simulink model "PPS_Scenario_003_cs"  (Simulink 7.6)
settings: Solver=ode5  SolverMode=SingleTasking  StartTime=0.0  StopTime=inf  FixedStep=1/100  RelTol=1e-3
model workspace (MAT data in the model file):
  mbox_table : struct (value not decoded)
  model_closed = 0
  sim_status = 0
PreLoadFcn:
  | check_NUTS_defined;
  | 
  | assignin('base',['model_closed_' bdroot],false);
  | 
  | addpath('../includes_PPS');
  | 
  | if exist('PPS_Model_sfun.mexw64')==3
  | delete PPS_Model_sfun.mexw64;
  | end
  | 
  | if exist('PPS_Model_sfun.mexw32') ==3
  | delete PPS_Model_sfun.mexw32;
  | end
  | 
  | switch version('-release')
  | case {'2010a', '2010b', '2011a'}
  | addpath('../includes_PPS/ML2010a');
  | case {'2011b', '2012a', '2012b'}
  | addpath('../includes_PPS/ML2011b');
  | otherwise
  | addpath('../includes_PPS/ML2011b');
  | end
InitFcn:
  | PreScanExperimentInitFcn(bdroot)
StopFcn:
  | PreScanExperimentStopFcn(bdroot)
undefined symbols (not defined in the file): DiscIntNeverNeededParam, InitImageOutputDir, x_ini_VRML, y_ini_VRML, z_ini_VRML
libraries: PreScanSimulinkLibrary x48, simulink x27, PreScanUsefulBlocks x20, simulink_extras x9, simulink_need_slupdate x1
(part 1 of 14)
CloseFcn:
  | evalin('base',['clear model_closed_' bdroot]);
settings Model: Creator=PRESCAN  LastModifiedBy=buildbot
settings DataIOCC: LimitDataPoints=off  MaxDataPoints=1  SaveOutput=off  SignalLogging=off  DSMLogging=off
settings OptimizationCC: InitFltsAndDblsToZero=on
settings DebuggingCC: SaveWithParameterizedLinksMsg=none  SignalResolutionControl=TryResolveAllWithWarning  SolverPrmCheckMsg=none  MultiTaskDSMMsg=warning  MultiTaskCondExecSysMsg=none  MultiTaskRateTransMsg=warning  UnknownTsInhSupMsg=none
settings SFSimCC: SimParseCustomCode=off
settings RTWCC: IncludeERTFirstTime=on
settings GRTTargetCC: TargetFcnLib=ansi_tfl_tmw.mat

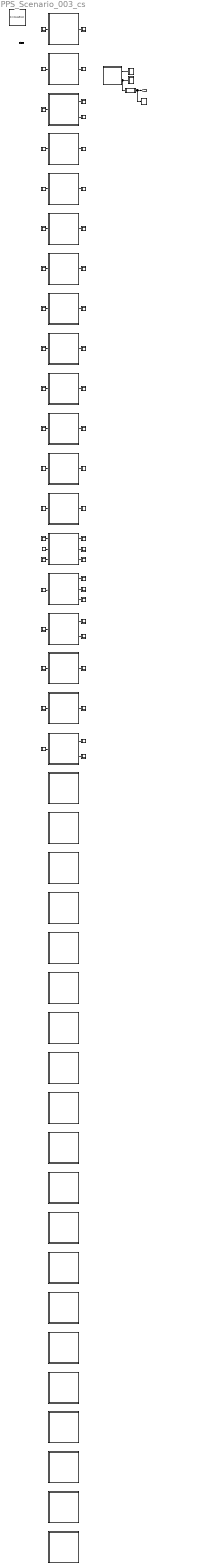
== system PPS_Scenario_003_cs ==
  note: OBU-Beacon ID
  note: Demo Help
  note: Regenerate
  note: Record for Replay
  note: Open Useful Blocks
  note: PreScan Options
  note: Version:
  note: 7.4.0
  note: Author(s):
  note: N.A.
  note: Descriptive text:
  note: ID
      |
      | 1
      | 8
      | 11
      | 16
      | 12
      | 19
      | 31
      | 47
      | 48
      | 49
      | 73
      | 93
      | 4
      | 7
      | 32
      | 66
      | 67
      | 68
      | 65
      | 15
      | 76
      | 10
      | 3
      | 78
      | 77
      | 79
      | 80
      | 81
      | 82
      | 83
      | 84
      | 85
      | 86
      | 89
      | 90
      | 92
      | 94
      | 95
      | 96
      | 103
      | 104
      | 105
      | 106
      | 114
      | 115
      | 57
      | 53
      | 58
      | 70
      | 97
      | 99
      | 100
      | 110
      | 108
      | 109
      | 112
  note: OBU-Beacon ID
  note: TypeID
      |
      | 1
      | 1
      | 1
      | 3
      | 4
      | 1
      | 1
      | 1
      | 1
      | 1
      | 3
      | 1
      | 1
      | 1
      | 1
      | 1
      | 7
      | 5
      | 1
      | 14
      | 14
      | 12
      | 12
      | 15
      | 15
      | 15
      | 15
      | 15
      | 15
      | 15
      | 15
      | 15
      | 15
      | 15
      | 15
      | 15
      | 15
      | 15
      | 15
      | 15
      | 15
      | 15
      | 15
      | 15
      | 15
      | 13
      | 13
      | 13
      | 13
      | 13
      | 13
      | 13
      | 13
      | 13
      | 13
      | 13
  note: TypeTag
      |
      | Car
      | Car
      | Car
      | Truck\Bus
      | Human
      | Car
      | Car
      | Car
      | Car
      | Car
      | Truck\Bus
      | Car
      | Car
      | Car
      | Car
      | Car
      | Unknown
      | Cal element
      | Car
      | Traffic sign
      | Traffic sign
      | Building
      | Building
      | Anim traffic sign
      | Anim traffic sign
      | Anim traffic sign
      | Anim traffic sign
      | Anim traffic sign
      | Anim traffic sign
      | Anim traffic sign
      | Anim traffic sign
      | Anim traffic sign
      | Anim traffic sign
      | Anim traffic sign
      | Anim traffic sign
      | Anim traffic sign
      | Anim traffic sign
      | Anim traffic sign
      | Anim traffic sign
      | Anim traffic sign
      | Anim traffic sign
      | Anim traffic sign
      | Anim traffic sign
      | Anim traffic sign
      | Anim traffic sign
      | Natural element
      | Natural element
      | Natural element
      | Natural element
      | Natural element
      | Natural element
      | Natural element
      | Natural element
      | Natural element
      | Natural element
      | Natural element
  note: SD
      |
      | Y
      | Y
      | Y
      | Y
      | Y
      | Y
      | Y
      | Y
      | Y
      | Y
      | Y
      | N
      | N
      | N
      | Y
      | Y
      | Y
      | Y
      | Y
      | Y
      | Y
      | Y
      | Y
      | Y
      | N
      | Y
      | Y
      | Y
      | Y
      | Y
      | Y
      | N
      | N
      | Y
      | Y
      | Y
      | Y
      | Y
      | Y
      | N
      | N
      | N
      | N
      | Y
      | Y
      | Y
      | Y
      | Y
      | Y
      | Y
      | Y
      | Y
      | Y
      | Y
      | Y
      | Y
  note: CD
      |
      | N
      | N
      | N
      | N
      | Y
      | N
      | N
      | N
      | N
      | N
      | N
      | N
      | N
      | Y
      | N
      | N
      | N
      | N
      | N
      | N
      | N
      | N
      | N
      | N
      | N
      | N
      | N
      | N
      | N
      | N
      | N
      | N
      | N
      | N
      | N
      | N
      | N
      | N
      | N
      | N
      | N
      | N
      | N
      | N
      | N
      | N
      | N
      | N
      | N
      | N
      | N
      | N
      | N
      | N
      | N
      | N
  note: Name
      |
      | BMW_X5_1
      | BMW_Z3_1
      | Toyota_Previa_1
      | Nissan_Cabstar_1
      | HumanAnimated_1
      | Mazda_RX8_2
      | Fiat_Bravo_2
      | Toyota_Previa_2
      | Toyota_Previa_3
      | Mazda_RX8_3
      | Nissan_Cabstar_2
      | Toyota_Previa_4
      | BMW_X5_2
      | Audi_A8_1
      | Toyota_Yaris_1
      | Ford_Fiesta_1
      | CarTrailer_SingleAxle_1
      | Sphere_1
      | Fiat_Bravo_1
      | TrafficSignPoleD_1
      | TrafficSignPoleD_2
      | OfficeBrownFlat_1
      | Busstop_1
      | Lightpost_2
      | Lightpost_1
      | Lightpost_3
      | Lightpost_4
      | Lightpost_5
      | Lightpost_6
      | Lightpost_7
      | Lightpost_8
      | Lightpost_9
      | Lightpost_10
      | InformationBoard_1
      | InformationBoard_2
      | Lightpost_11
      | Lightpost_12
      | Lightpost_13
      | Lightpost_14
      | Lightpost_15
      | Lightpost_16
      | Lightpost_17
      | Lightpost_18
      | Lightpost_19
      | Lightpost_20
      | TurkishHazel_Age20_5
      | TurkishHazel_Age10_1
      | TurkishHazel_Age10_2
      | TurkishHazel_Age20_1
      | TurkishHazel_Age20_6
      | TurkishHazel_Age20_8
      | TurkishHazel_Age20_9
      | TurkishHazel_Age20_13
      | TurkishHazel_Age20_10
      | TurkishHazel_Age20_11
      | TurkishHazel_Age20_12
  note: Num ID OBU-Beacon ID Type ID Type Tag SD CD Name
  Actuators : DataStoreMemory  Tag=Actuators  DataStoreName=SimCoreActuators  InitialValue=zeros(572,1)
      settings: DeleteFcn=PreScanBlockDeleteFcn;
  Audi_A8_1 : Subsystem  Tag=WorldObjectSubSystem  InitFcn=UniqueId = '210';
      mask Display: image(imread('Audi_A8.jpg'));color('white');text(0,0,' ID=7\n')
  BMW_X5_1 : Subsystem  Tag=WorldObjectSubSystem  InitFcn=UniqueId = '19';
      mask Display: image(imread('BMW_X5.jpg'));color('white');text(0,0,' ID=1\n')
  BMW_X5_2 : Subsystem  Tag=WorldObjectSubSystem  InitFcn=UniqueId = '173';
      mask Display: image(imread('BMW_X5.jpg'));color('white');text(0,0,' ID=4\n')
  BMW_Z3_1 : Subsystem  Tag=WorldObjectSubSystem  InitFcn=UniqueId = '21';
      mask Display: image(imread('BMW_Z3.jpg'));color('white');text(0,0,' ID=8\n')
  CameraSensor_1 : Subsystem  Tag=CameraSensor  Priority=3
      settings: DeleteFcn=PreScanBlockDeleteFcn;
      mask Type: PreScan Source Block: Camera Sensor
      mask Description: The Camera Sensor provides a color or monochrome image.
      mask Help: eval('openHelp(457)')
      mask Display: image(imread('CameraSensor.png'))
  CarTrailer_SingleAxle_1 : Subsystem  Tag=WorldObjectSubSystem  InitFcn=UniqueId = '232';
      mask Display: image(imread('CarTrailer_SingleAxle.jpg'));color('white');text(0,0,' ID=67\n')
  CollisionDetection : Subsystem  Tag=CollisionDetection  Priority=3  mask(PreScan Source Block: CollisionDetection){PortName=CollisionDetection, PortIndex=0, PortWidth=10, TimeStep=1/100}
      mask prompts: PortName "Auto-Assigned: Port Name [-]"; PortIndex "Auto-Assigned: Port Index [-]"; PortWidth "Auto-Assigned: Port Dimensions"; TimeStep "Auto-Assigned: Upload Period [s]"
      mask help:
      | The SELF port shows (state) information of the actor itself. The outputs are position in the experiment's axis system and the GPS coordinates, and the object's absolute velocity and compass heading.
      |
      | For more information, please click Help.
      settings: DeleteFcn=PreScanBlockDeleteFcn;
      mask Help: eval('openHelp(811)')
      mask Display: image(imread('crash.jpg'))
  Fiat_Bravo_1 : Subsystem  Tag=WorldObjectSubSystem  InitFcn=UniqueId = '271';
      mask Display: image(imread('Fiat_Bravo.jpg'));color('white');text(0,0,' ID=65\n')
  Fiat_Bravo_2 : Subsystem  Tag=WorldObjectSubSystem  InitFcn=UniqueId = '139';
      mask Display: image(imread('Fiat_Bravo.jpg'));color('white');text(0,0,' ID=31\n')
  Ford_Fiesta_1 : Subsystem  Tag=WorldObjectSubSystem  InitFcn=UniqueId = '231';
      mask Display: image(imread('Ford_Fiesta.jpg'));color('white');text(0,0,' ID=66\n')
  GetSensors : Subsystem  Tag=GetSensors  Priority=2  mask(PreScan Simulation Core Block){NrOfSensors=162, TimeStep=1/100}
      mask prompts: NrOfSensors "Number of sensor values"; TimeStep "Timestep [s]"
      mask help:
      | Please do not remove this block from the PreScan compilation sheet,
      | as it contains essential configuration parameters for a PreScan simulation.
      settings: DeleteFcn=PreScanBlockDeleteFcn;
  HumanAnimated_1 : Subsystem  Tag=WorldObjectSubSystem  InitFcn=UniqueId = '71';
      mask Display: image(imread('HumanTextured.jpg'));color('white');text(0,0,' ID=12\n')
  Lightpost_1 : Subsystem  Tag=WorldObjectSubSystem  InitFcn=UniqueId = '149';
      mask Display: image(imread('Lightpost.jpg'));color('white');text(0,0,' ID=77\n')
  Lightpost_10 : Subsystem  Tag=WorldObjectSubSystem  InitFcn=UniqueId = '157';
      mask Display: image(imread('Lightpost.jpg'));color('white');text(0,0,' ID=86\n')
  Lightpost_11 : Subsystem  Tag=WorldObjectSubSystem  InitFcn=UniqueId = '254';
      mask Display: image(imread('Lightpost.jpg'));color('white');text(0,0,' ID=92\n')
  Lightpost_12 : Subsystem  Tag=WorldObjectSubSystem  InitFcn=UniqueId = '256';
      mask Display: image(imread('Lightpost.jpg'));color('white');text(0,0,' ID=94\n')
  Lightpost_13 : Subsystem  Tag=WorldObjectSubSystem  InitFcn=UniqueId = '257';
      mask Display: image(imread('Lightpost.jpg'));color('white');text(0,0,' ID=95\n')
  Lightpost_14 : Subsystem  Tag=WorldObjectSubSystem  InitFcn=UniqueId = '258';
      mask Display: image(imread('Lightpost.jpg'));color('white');text(0,0,' ID=96\n')
  Lightpost_15 : Subsystem  Tag=WorldObjectSubSystem  InitFcn=UniqueId = '274';
      mask Display: image(imread('Lightpost.jpg'));color('white');text(0,0,' ID=103\n')
  Lightpost_16 : Subsystem  Tag=WorldObjectSubSystem  InitFcn=UniqueId = '275';
      mask Display: image(imread('Lightpost.jpg'));color('white');text(0,0,' ID=104\n')
  Lightpost_17 : Subsystem  Tag=WorldObjectSubSystem  InitFcn=UniqueId = '276';
      mask Display: image(imread('Lightpost.jpg'));color('white');text(0,0,' ID=105\n')
  Lightpost_18 : Subsystem  Tag=WorldObjectSubSystem  InitFcn=UniqueId = '277';
      mask Display: image(imread('Lightpost.jpg'));color('white');text(0,0,' ID=106\n')
  Lightpost_19 : Subsystem  Tag=WorldObjectSubSystem  InitFcn=UniqueId = '290';
      mask Display: image(imread('Lightpost.jpg'));color('white');text(0,0,' ID=114\n')
  Lightpost_2 : Subsystem  Tag=WorldObjectSubSystem  InitFcn=UniqueId = '148';
      mask Display: image(imread('Lightpost.jpg'));color('white');text(0,0,' ID=78\n')
  Lightpost_20 : Subsystem  Tag=WorldObjectSubSystem  InitFcn=UniqueId = '291';
      mask Display: image(imread('Lightpost.jpg'));color('white');text(0,0,' ID=115\n')
  Lightpost_3 : Subsystem  Tag=WorldObjectSubSystem  InitFcn=UniqueId = '150';
      mask Display: image(imread('Lightpost.jpg'));color('white');text(0,0,' ID=79\n')
  Lightpost_4 : Subsystem  Tag=WorldObjectSubSystem  InitFcn=UniqueId = '151';
      mask Display: image(imread('Lightpost.jpg'));color('white');text(0,0,' ID=80\n')
  Lightpost_5 : Subsystem  Tag=WorldObjectSubSystem  InitFcn=UniqueId = '152';
      mask Display: image(imread('Lightpost.jpg'));color('white');text(0,0,' ID=81\n')
  Lightpost_6 : Subsystem  Tag=WorldObjectSubSystem  InitFcn=UniqueId = '153';
      mask Display: image(imread('Lightpost.jpg'));color('white');text(0,0,' ID=82\n')
  Lightpost_7 : Subsystem  Tag=WorldObjectSubSystem  InitFcn=UniqueId = '154';
      mask Display: image(imread('Lightpost.jpg'));color('white');text(0,0,' ID=83\n')
  Lightpost_8 : Subsystem  Tag=WorldObjectSubSystem  InitFcn=UniqueId = '155';
      mask Display: image(imread('Lightpost.jpg'));color('white');text(0,0,' ID=84\n')
  Lightpost_9 : Subsystem  Tag=WorldObjectSubSystem  InitFcn=UniqueId = '156';
      mask Display: image(imread('Lightpost.jpg'));color('white');text(0,0,' ID=85\n')
  Mazda_RX8_2 : Subsystem  Tag=WorldObjectSubSystem  InitFcn=UniqueId = '114';
      mask Display: image(imread('Mazda_RX8.jpg'));color('white');text(0,0,' ID=19\n')
  Mazda_RX8_3 : Subsystem  Tag=WorldObjectSubSystem  InitFcn=UniqueId = '143';
      mask Display: image(imread('Mazda_RX8.jpg'));color('white');text(0,0,' ID=49\n')
  Nissan_Cabstar_1 : Subsystem  Tag=WorldObjectSubSystem  InitFcn=UniqueId = '45';
      mask Display: image(imread('Nissan_Cabstar.jpg'));color('white');text(0,0,' ID=16\n')
  Nissan_Cabstar_2 : Subsystem  Tag=WorldObjectSubSystem  InitFcn=UniqueId = '144';
      mask Display: image(imread('Nissan_Cabstar.jpg'));color('white');text(0,0,' ID=73\n')
  SELF_Audi_A8_1 : Subsystem  Tag=SELF  Priority=3  mask(PreScan Source Block: SELF){PortName=SELF_Audi_A8_1, PortIndex=114, PortWidth=8, TimeStep=1/100}
      mask prompts: PortName "Auto-Assigned: Port Name [-]"; PortIndex "Auto-Assigned: Port Index [-]"; PortWidth "Auto-Assigned: Port Dimensions"; TimeStep "Auto-Assigned: Upload Period [s]"
      mask help:
      | The SELF port shows (state) information of the actor itself. The outputs are position in the experiment's axis system and the GPS coordinates, and the object's absolute velocity and compass heading.
      |
      | For more information, please click Help.
      settings: DeleteFcn=PreScanBlockDeleteFcn;
      mask Help: eval('openHelp(462)')
      mask Display: image(imread('GPS.png'))
  SELF_BMW_X5_1 : Subsystem  Tag=SELF  Priority=3  mask(PreScan Source Block: SELF){PortName=SELF_BMW_X5_1, PortIndex=10, PortWidth=8, TimeStep=1/100}
      mask prompts: PortName "Auto-Assigned: Port Name [-]"; PortIndex "Auto-Assigned: Port Index [-]"; PortWidth "Auto-Assigned: Port Dimensions"; TimeStep "Auto-Assigned: Upload Period [s]"
      mask help:
      | The SELF port shows (state) information of the actor itself. The outputs are position in the experiment's axis system and the GPS coordinates, and the object's absolute velocity and compass heading.
      |
      | For more information, please click Help.
      settings: DeleteFcn=PreScanBlockDeleteFcn;
      mask Help: eval('openHelp(462)')
      mask Display: image(imread('GPS.png'))
  SELF_BMW_X5_2 : Subsystem  Tag=SELF  Priority=3  mask(PreScan Source Block: SELF){PortName=SELF_BMW_X5_2, PortIndex=106, PortWidth=8, TimeStep=1/100}
      mask prompts: PortName "Auto-Assigned: Port Name [-]"; PortIndex "Auto-Assigned: Port Index [-]"; PortWidth "Auto-Assigned: Port Dimensions"; TimeStep "Auto-Assigned: Upload Period [s]"
      mask help:
      | The SELF port shows (state) information of the actor itself. The outputs are position in the experiment's axis system and the GPS coordinates, and the object's absolute velocity and compass heading.
      |
      | For more information, please click Help.
      settings: DeleteFcn=PreScanBlockDeleteFcn;
      mask Help: eval('openHelp(462)')
      mask Display: image(imread('GPS.png'))
  SELF_BMW_Z3_1 : Subsystem  Tag=SELF  Priority=3  mask(PreScan Source Block: SELF){PortName=SELF_BMW_Z3_1, PortIndex=18, PortWidth=8, TimeStep=1/100}
      mask prompts: PortName "Auto-Assigned: Port Name [-]"; PortIndex "Auto-Assigned: Port Index [-]"; PortWidth "Auto-Assigned: Port Dimensions"; TimeStep "Auto-Assigned: Upload Period [s]"
      mask help:
      | The SELF port shows (state) information of the actor itself. The outputs are position in the experiment's axis system and the GPS coordinates, and the object's absolute velocity and compass heading.
      |
      | For more information, please click Help.
      settings: DeleteFcn=PreScanBlockDeleteFcn;
      mask Help: eval('openHelp(462)')
      mask Display: image(imread('GPS.png'))
  SELF_CarTrailer_SingleAxle_1 : Subsystem  Tag=SELF  Priority=3  mask(PreScan Source Block: SELF){PortName=SELF_CarTrailer_SingleAxle_1, PortIndex=138, PortWidth=8, TimeStep=1/100}
      mask prompts: PortName "Auto-Assigned: Port Name [-]"; PortIndex "Auto-Assigned: Port Index [-]"; PortWidth "Auto-Assigned: Port Dimensions"; TimeStep "Auto-Assigned: Upload Period [s]"
      mask help:
      | The SELF port shows (state) information of the actor itself. The outputs are position in the experiment's axis system and the GPS coordinates, and the object's absolute velocity and compass heading.
      |
      | For more information, please click Help.
      settings: DeleteFcn=PreScanBlockDeleteFcn;
      mask Help: eval('openHelp(462)')
      mask Display: image(imread('GPS.png'))
  SELF_Fiat_Bravo_1 : Subsystem  Tag=SELF  Priority=3  mask(PreScan Source Block: SELF){PortName=SELF_Fiat_Bravo_1, PortIndex=154, PortWidth=8, TimeStep=1/100}
      mask prompts: PortName "Auto-Assigned: Port Name [-]"; PortIndex "Auto-Assigned: Port Index [-]"; PortWidth "Auto-Assigned: Port Dimensions"; TimeStep "Auto-Assigned: Upload Period [s]"
      mask help:
      | The SELF port shows (state) information of the actor itself. The outputs are position in the experiment's axis system and the GPS coordinates, and the object's absolute velocity and compass heading.
      |
      | For more information, please click Help.
      settings: DeleteFcn=PreScanBlockDeleteFcn;
      mask Help: eval('openHelp(462)')
      mask Display: image(imread('GPS.png'))
  SELF_Fiat_Bravo_2 : Subsystem  Tag=SELF  Priority=3  mask(PreScan Source Block: SELF){PortName=SELF_Fiat_Bravo_2, PortIndex=58, PortWidth=8, TimeStep=1/100}
      mask prompts: PortName "Auto-Assigned: Port Name [-]"; PortIndex "Auto-Assigned: Port Index [-]"; PortWidth "Auto-Assigned: Port Dimensions"; TimeStep "Auto-Assigned: Upload Period [s]"
      mask help:
      | The SELF port shows (state) information of the actor itself. The outputs are position in the experiment's axis system and the GPS coordinates, and the object's absolute velocity and compass heading.
      |
      | For more information, please click Help.
      settings: DeleteFcn=PreScanBlockDeleteFcn;
      mask Help: eval('openHelp(462)')
      mask Display: image(imread('GPS.png'))
  SELF_Ford_Fiesta_1 : Subsystem  Tag=SELF  Priority=3  mask(PreScan Source Block: SELF){PortName=SELF_Ford_Fiesta_1, PortIndex=130, PortWidth=8, TimeStep=1/100}
      mask prompts: PortName "Auto-Assigned: Port Name [-]"; PortIndex "Auto-Assigned: Port Index [-]"; PortWidth "Auto-Assigned: Port Dimensions"; TimeStep "Auto-Assigned: Upload Period [s]"
      mask help:
      | The SELF port shows (state) information of the actor itself. The outputs are position in the experiment's axis system and the GPS coordinates, and the object's absolute velocity and compass heading.
      |
      | For more information, please click Help.
      settings: DeleteFcn=PreScanBlockDeleteFcn;
      mask Help: eval('openHelp(462)')
      mask Display: image(imread('GPS.png'))
  SELF_HumanAnimated_1 : Subsystem  Tag=SELF  Priority=3  mask(PreScan Source Block: SELF){PortName=SELF_HumanAnimated_1, PortIndex=42, PortWidth=8, TimeStep=1/100}
      mask prompts: PortName "Auto-Assigned: Port Name [-]"; PortIndex "Auto-Assigned: Port Index [-]"; PortWidth "Auto-Assigned: Port Dimensions"; TimeStep "Auto-Assigned: Upload Period [s]"
      mask help:
      | The SELF port shows (state) information of the actor itself. The outputs are position in the experiment's axis system and the GPS coordinates, and the object's absolute velocity and compass heading.
      |
      | For more information, please click Help.
      settings: DeleteFcn=PreScanBlockDeleteFcn;
      mask Help: eval('openHelp(462)')
      mask Display: image(imread('GPS.png'))
  SELF_Mazda_RX8_2 : Subsystem  Tag=SELF  Priority=3  mask(PreScan Source Block: SELF){PortName=SELF_Mazda_RX8_2, PortIndex=50, PortWidth=8, TimeStep=1/100}
      mask prompts: PortName "Auto-Assigned: Port Name [-]"; PortIndex "Auto-Assigned: Port Index [-]"; PortWidth "Auto-Assigned: Port Dimensions"; TimeStep "Auto-Assigned: Upload Period [s]"
      mask help:
      | The SELF port shows (state) information of the actor itself. The outputs are position in the experiment's axis system and the GPS coordinates, and the object's absolute velocity and compass heading.
      |
      | For more information, please click Help.
      settings: DeleteFcn=PreScanBlockDeleteFcn;
      mask Help: eval('openHelp(462)')
      mask Display: image(imread('GPS.png'))
  SELF_Mazda_RX8_3 : Subsystem  Tag=SELF  Priority=3  mask(PreScan Source Block: SELF){PortName=SELF_Mazda_RX8_3, PortIndex=82, PortWidth=8, TimeStep=1/100}
      mask prompts: PortName "Auto-Assigned: Port Name [-]"; PortIndex "Auto-Assigned: Port Index [-]"; PortWidth "Auto-Assigned: Port Dimensions"; TimeStep "Auto-Assigned: Upload Period [s]"
      mask help:
      | The SELF port shows (state) information of the actor itself. The outputs are position in the experiment's axis system and the GPS coordinates, and the object's absolute velocity and compass heading.
      |
      | For more information, please click Help.
      settings: DeleteFcn=PreScanBlockDeleteFcn;
      mask Help: eval('openHelp(462)')
      mask Display: image(imread('GPS.png'))
  SELF_Nissan_Cabstar_1 : Subsystem  Tag=SELF  Priority=3  mask(PreScan Source Block: SELF){PortName=SELF_Nissan_Cabstar_1, PortIndex=34, PortWidth=8, TimeStep=1/100}
      mask prompts: PortName "Auto-Assigned: Port Name [-]"; PortIndex "Auto-Assigned: Port Index [-]"; PortWidth "Auto-Assigned: Port Dimensions"; TimeStep "Auto-Assigned: Upload Period [s]"
      mask help:
      | The SELF port shows (state) information of the actor itself. The outputs are position in the experiment's axis system and the GPS coordinates, and the object's absolute velocity and compass heading.
      |
      | For more information, please click Help.
      settings: DeleteFcn=PreScanBlockDeleteFcn;
      mask Help: eval('openHelp(462)')
      mask Display: image(imread('GPS.png'))
  SELF_Nissan_Cabstar_2 : Subsystem  Tag=SELF  Priority=3  mask(PreScan Source Block: SELF){PortName=SELF_Nissan_Cabstar_2, PortIndex=90, PortWidth=8, TimeStep=1/100}
      mask prompts: PortName "Auto-Assigned: Port Name [-]"; PortIndex "Auto-Assigned: Port Index [-]"; PortWidth "Auto-Assigned: Port Dimensions"; TimeStep "Auto-Assigned: Upload Period [s]"
      mask help:
      | The SELF port shows (state) information of the actor itself. The outputs are position in the experiment's axis system and the GPS coordinates, and the object's absolute velocity and compass heading.
      |
      | For more information, please click Help.
      settings: DeleteFcn=PreScanBlockDeleteFcn;
      mask Help: eval('openHelp(462)')
      mask Display: image(imread('GPS.png'))
  SELF_Sphere_1 : Subsystem  Tag=SELF  Priority=3  mask(PreScan Source Block: SELF){PortName=SELF_Sphere_1, PortIndex=146, PortWidth=8, TimeStep=1/100}
      mask prompts: PortName "Auto-Assigned: Port Name [-]"; PortIndex "Auto-Assigned: Port Index [-]"; PortWidth "Auto-Assigned: Port Dimensions"; TimeStep "Auto-Assigned: Upload Period [s]"
      mask help:
      | The SELF port shows (state) information of the actor itself. The outputs are position in the experiment's axis system and the GPS coordinates, and the object's absolute velocity and compass heading.
      |
      | For more information, please click Help.
      settings: DeleteFcn=PreScanBlockDeleteFcn;
      mask Help: eval('openHelp(462)')
      mask Display: image(imread('GPS.png'))
  SELF_Toyota_Previa_1 : Subsystem  Tag=SELF  Priority=3  mask(PreScan Source Block: SELF){PortName=SELF_Toyota_Previa_1, PortIndex=26, PortWidth=8, TimeStep=1/100}
      mask prompts: PortName "Auto-Assigned: Port Name [-]"; PortIndex "Auto-Assigned: Port Index [-]"; PortWidth "Auto-Assigned: Port Dimensions"; TimeStep "Auto-Assigned: Upload Period [s]"
      mask help:
      | The SELF port shows (state) information of the actor itself. The outputs are position in the experiment's axis system and the GPS coordinates, and the object's absolute velocity and compass heading.
      |
      | For more information, please click Help.
      settings: DeleteFcn=PreScanBlockDeleteFcn;
      mask Help: eval('openHelp(462)')
      mask Display: image(imread('GPS.png'))
  SELF_Toyota_Previa_2 : Subsystem  Tag=SELF  Priority=3  mask(PreScan Source Block: SELF){PortName=SELF_Toyota_Previa_2, PortIndex=66, PortWidth=8, TimeStep=1/100}
      mask prompts: PortName "Auto-Assigned: Port Name [-]"; PortIndex "Auto-Assigned: Port Index [-]"; PortWidth "Auto-Assigned: Port Dimensions"; TimeStep "Auto-Assigned: Upload Period [s]"
      mask help:
      | The SELF port shows (state) information of the actor itself. The outputs are position in the experiment's axis system and the GPS coordinates, and the object's absolute velocity and compass heading.
      |
      | For more information, please click Help.
      settings: DeleteFcn=PreScanBlockDeleteFcn;
      mask Help: eval('openHelp(462)')
      mask Display: image(imread('GPS.png'))
  SELF_Toyota_Previa_3 : Subsystem  Tag=SELF  Priority=3  mask(PreScan Source Block: SELF){PortName=SELF_Toyota_Previa_3, PortIndex=74, PortWidth=8, TimeStep=1/100}
      mask prompts: PortName "Auto-Assigned: Port Name [-]"; PortIndex "Auto-Assigned: Port Index [-]"; PortWidth "Auto-Assigned: Port Dimensions"; TimeStep "Auto-Assigned: Upload Period [s]"
      mask help:
      | The SELF port shows (state) information of the actor itself. The outputs are position in the experiment's axis system and the GPS coordinates, and the object's absolute velocity and compass heading.
      |
      | For more information, please click Help.
      settings: DeleteFcn=PreScanBlockDeleteFcn;
      mask Help: eval('openHelp(462)')
      mask Display: image(imread('GPS.png'))
  SELF_Toyota_Previa_4 : Subsystem  Tag=SELF  Priority=3  mask(PreScan Source Block: SELF){PortName=SELF_Toyota_Previa_4, PortIndex=98, PortWidth=8, TimeStep=1/100}
      mask prompts: PortName "Auto-Assigned: Port Name [-]"; PortIndex "Auto-Assigned: Port Index [-]"; PortWidth "Auto-Assigned: Port Dimensions"; TimeStep "Auto-Assigned: Upload Period [s]"
      mask help:
      | The SELF port shows (state) information of the actor itself. The outputs are position in the experiment's axis system and the GPS coordinates, and the object's absolute velocity and compass heading.
      |
      | For more information, please click Help.
      settings: DeleteFcn=PreScanBlockDeleteFcn;
      mask Help: eval('openHelp(462)')
      mask Display: image(imread('GPS.png'))
  SELF_Toyota_Yaris_1 : Subsystem  Tag=SELF  Priority=3  mask(PreScan Source Block: SELF){PortName=SELF_Toyota_Yaris_1, PortIndex=122, PortWidth=8, TimeStep=1/100}
      mask prompts: PortName "Auto-Assigned: Port Name [-]"; PortIndex "Auto-Assigned: Port Index [-]"; PortWidth "Auto-Assigned: Port Dimensions"; TimeStep "Auto-Assigned: Upload Period [s]"
      mask help:
      | The SELF port shows (state) information of the actor itself. The outputs are position in the experiment's axis system and the GPS coordinates, and the object's absolute velocity and compass heading.
      |
      | For more information, please click Help.
      settings: DeleteFcn=PreScanBlockDeleteFcn;
      mask Help: eval('openHelp(462)')
      mask Display: image(imread('GPS.png'))
  STATE_Audi_A8_1 : Subsystem  Tag=State  Priority=0  mask(PreScan Sink Block: State){x0=134.49999618530273, y0=66.661239624023438, z0=0.55, Roll0=0, Pitch0=0, Yaw0=180, TimeStep=1/100}
      mask prompts: x0 "Ini x-position VEHICLE wrt GLOBAL axis system [m]"; y0 "Ini y-position VEHICLE wrt GLOBAL axis system [m]"; z0 "Ini z-position VEHICLE wrt GLOBAL axis system [m]"; Roll0 "Ini roll-angle BODY wrt VEHICLE axis system [deg]"; Pitch0 "Ini pitch-angle BODY wrt VEHICLE axis system [deg]"; Yaw0 "Ini yaw-angle VEHICLE wrt GLOBAL axis system [deg]"; TimeStep "Time Step [s]"
      mask help:
      | The Actor State contains a vector signal of size (9x1), containing the following signals:
      |
      | -  Position                  (x,y,z)                                     [m]
      | -  Velocity                  (vx,vy,vz)                               [m/s]
      | -  Angles                    (Roll, Pitch, Yaw)                   [rad]
      |
      | The Actor state is defined in the global axis system.
      | The state is superponed on the Initial position defined in the GUI.
      |
      | For more information, please click Help.
      settings: DeleteFcn=PreScanBlockDeleteFcn;
      mask Help: eval('openHelp(222)')
      mask Display: image(imread('State.png'))
  STATE_BMW_X5_1 : Subsystem  Tag=State  Priority=0  mask(PreScan Sink Block: State){x0=121.58638000488281, y0=70.2, z0=0.68999999761581421, Roll0=0, Pitch0=0, Yaw0=180, TimeStep=1/100}
      mask prompts: x0 "Ini x-position VEHICLE wrt GLOBAL axis system [m]"; y0 "Ini y-position VEHICLE wrt GLOBAL axis system [m]"; z0 "Ini z-position VEHICLE wrt GLOBAL axis system [m]"; Roll0 "Ini roll-angle BODY wrt VEHICLE axis system [deg]"; Pitch0 "Ini pitch-angle BODY wrt VEHICLE axis system [deg]"; Yaw0 "Ini yaw-angle VEHICLE wrt GLOBAL axis system [deg]"; TimeStep "Time Step [s]"
      mask help:
      | The Actor State contains a vector signal of size (9x1), containing the following signals:
      |
      | -  Position                  (x,y,z)                                     [m]
      | -  Velocity                  (vx,vy,vz)                               [m/s]
      | -  Angles                    (Roll, Pitch, Yaw)                   [rad]
      |
      | The Actor state is defined in the global axis system.
      | The state is superponed on the Initial position defined in the GUI.
      |
      | For more information, please click Help.
      settings: DeleteFcn=PreScanBlockDeleteFcn;
      mask Help: eval('openHelp(222)')
      mask Display: image(imread('State.png'))
  STATE_BMW_X5_2 : Subsystem  Tag=State  Priority=0  mask(PreScan Sink Block: State){x0=118.86122894287109, y0=90.418052673339844, z0=0.68999999761581421, Roll0=0, Pitch0=0, Yaw0=90, TimeStep=1/100}
      mask prompts: x0 "Ini x-position VEHICLE wrt GLOBAL axis system [m]"; y0 "Ini y-position VEHICLE wrt GLOBAL axis system [m]"; z0 "Ini z-position VEHICLE wrt GLOBAL axis system [m]"; Roll0 "Ini roll-angle BODY wrt VEHICLE axis system [deg]"; Pitch0 "Ini pitch-angle BODY wrt VEHICLE axis system [deg]"; Yaw0 "Ini yaw-angle VEHICLE wrt GLOBAL axis system [deg]"; TimeStep "Time Step [s]"
      mask help:
      | The Actor State contains a vector signal of size (9x1), containing the following signals:
      |
      | -  Position                  (x,y,z)                                     [m]
      | -  Velocity                  (vx,vy,vz)                               [m/s]
      | -  Angles                    (Roll, Pitch, Yaw)                   [rad]
      |
      | The Actor state is defined in the global axis system.
      | The state is superponed on the Initial position defined in the GUI.
      |
      | For more information, please click Help.
      settings: DeleteFcn=PreScanBlockDeleteFcn;
      mask Help: eval('openHelp(222)')
      mask Display: image(imread('State.png'))
  STATE_BMW_Z3_1 : Subsystem  Tag=State  Priority=0  mask(PreScan Sink Block: State){x0=93.8578872680664, y0=70.123377990722659, z0=0.68999999761581421, Roll0=0, Pitch0=0, Yaw0=180, TimeStep=1/100}
      mask prompts: x0 "Ini x-position VEHICLE wrt GLOBAL axis system [m]"; y0 "Ini y-position VEHICLE wrt GLOBAL axis system [m]"; z0 "Ini z-position VEHICLE wrt GLOBAL axis system [m]"; Roll0 "Ini roll-angle BODY wrt VEHICLE axis system [deg]"; Pitch0 "Ini pitch-angle BODY wrt VEHICLE axis system [deg]"; Yaw0 "Ini yaw-angle VEHICLE wrt GLOBAL axis system [deg]"; TimeStep "Time Step [s]"
      mask help:
      | The Actor State contains a vector signal of size (9x1), containing the following signals:
      |
      | -  Position                  (x,y,z)                                     [m]
      | -  Velocity                  (vx,vy,vz)                               [m/s]
      | -  Angles                    (Roll, Pitch, Yaw)                   [rad]
      |
      | The Actor state is defined in the global axis system.
      | The state is superponed on the Initial position defined in the GUI.
      |
      | For more information, please click Help.
      settings: DeleteFcn=PreScanBlockDeleteFcn;
      mask Help: eval('openHelp(222)')
      mask Display: image(imread('State.png'))
  STATE_CarTrailer_SingleAxle_1 : Subsystem  Tag=State  Priority=0  mask(PreScan Sink Block: State){x0=53.920000000000009, y0=59.661239624023445, z0=0.45, Roll0=0, Pitch0=0, Yaw0=0, TimeStep=1/100}
      mask prompts: x0 "Ini x-position VEHICLE wrt GLOBAL axis system [m]"; y0 "Ini y-position VEHICLE wrt GLOBAL axis system [m]"; z0 "Ini z-position VEHICLE wrt GLOBAL axis system [m]"; Roll0 "Ini roll-angle BODY wrt VEHICLE axis system [deg]"; Pitch0 "Ini pitch-angle BODY wrt VEHICLE axis system [deg]"; Yaw0 "Ini yaw-angle VEHICLE wrt GLOBAL axis system [deg]"; TimeStep "Time Step [s]"
      mask help:
      | The Actor State contains a vector signal of size (9x1), containing the following signals:
      |
      | -  Position                  (x,y,z)                                     [m]
      | -  Velocity                  (vx,vy,vz)                               [m/s]
      | -  Angles                    (Roll, Pitch, Yaw)                   [rad]
      |
      | The Actor state is defined in the global axis system.
      | The state is superponed on the Initial position defined in the GUI.
      |
      | For more information, please click Help.
      settings: DeleteFcn=PreScanBlockDeleteFcn;
      mask Help: eval('openHelp(222)')
      mask Display: image(imread('State.png'))
  STATE_Fiat_Bravo_1 : Subsystem  Tag=State  Priority=0  mask(PreScan Sink Block: State){x0=149.8, y0=70.2, z0=0.55, Roll0=0, Pitch0=0, Yaw0=180, TimeStep=1/100}
      mask prompts: x0 "Ini x-position VEHICLE wrt GLOBAL axis system [m]"; y0 "Ini y-position VEHICLE wrt GLOBAL axis system [m]"; z0 "Ini z-position VEHICLE wrt GLOBAL axis system [m]"; Roll0 "Ini roll-angle BODY wrt VEHICLE axis system [deg]"; Pitch0 "Ini pitch-angle BODY wrt VEHICLE axis system [deg]"; Yaw0 "Ini yaw-angle VEHICLE wrt GLOBAL axis system [deg]"; TimeStep "Time Step [s]"
      mask help:
      | The Actor State contains a vector signal of size (9x1), containing the following signals:
      |
      | -  Position                  (x,y,z)                                     [m]
      | -  Velocity                  (vx,vy,vz)                               [m/s]
      | -  Angles                    (Roll, Pitch, Yaw)                   [rad]
      |
      | The Actor state is defined in the global axis system.
      | The state is superponed on the Initial position defined in the GUI.
      |
      | For more information, please click Help.
      settings: DeleteFcn=PreScanBlockDeleteFcn;
      mask Help: eval('openHelp(222)')
      mask Display: image(imread('State.png'))
  STATE_Fiat_Bravo_2 : Subsystem  Tag=State  Priority=0  mask(PreScan Sink Block: State){x0=101.32407379150391, y0=52.638362884521484, z0=0.57999998331069946, Roll0=0, Pitch0=0, Yaw0=0, TimeStep=1/100}
      mask prompts: x0 "Ini x-position VEHICLE wrt GLOBAL axis system [m]"; y0 "Ini y-position VEHICLE wrt GLOBAL axis system [m]"; z0 "Ini z-position VEHICLE wrt GLOBAL axis system [m]"; Roll0 "Ini roll-angle BODY wrt VEHICLE axis system [deg]"; Pitch0 "Ini pitch-angle BODY wrt VEHICLE axis system [deg]"; Yaw0 "Ini yaw-angle VEHICLE wrt GLOBAL axis system [deg]"; TimeStep "Time Step [s]"
      mask help:
      | The Actor State contains a vector signal of size (9x1), containing the following signals:
      |
      | -  Position                  (x,y,z)                                     [m]
      | -  Velocity                  (vx,vy,vz)                               [m/s]
      | -  Angles                    (Roll, Pitch, Yaw)                   [rad]
      |
      | The Actor state is defined in the global axis system.
      | The state is superponed on the Initial position defined in the GUI.
      |
      | For more information, please click Help.
      settings: DeleteFcn=PreScanBlockDeleteFcn;
      mask Help: eval('openHelp(222)')
      mask Display: image(imread('State.png'))
  STATE_Ford_Fiesta_1 : Subsystem  Tag=State  Priority=0  mask(PreScan Sink Block: State){x0=56.000000000000007, y0=59.661239624023445, z0=0.55, Roll0=0, Pitch0=0, Yaw0=0, TimeStep=1/100}
      mask prompts: x0 "Ini x-position VEHICLE wrt GLOBAL axis system [m]"; y0 "Ini y-position VEHICLE wrt GLOBAL axis system [m]"; z0 "Ini z-position VEHICLE wrt GLOBAL axis system [m]"; Roll0 "Ini roll-angle BODY wrt VEHICLE axis system [deg]"; Pitch0 "Ini pitch-angle BODY wrt VEHICLE axis system [deg]"; Yaw0 "Ini yaw-angle VEHICLE wrt GLOBAL axis system [deg]"; TimeStep "Time Step [s]"
      mask help:
      | The Actor State contains a vector signal of size (9x1), containing the following signals:
      |
      | -  Position                  (x,y,z)                                     [m]
      | -  Velocity                  (vx,vy,vz)                               [m/s]
      | -  Angles                    (Roll, Pitch, Yaw)                   [rad]
      |
      | The Actor state is defined in the global axis system.
      | The state is superponed on the Initial position defined in the GUI.
      |
      | For more information, please click Help.
      settings: DeleteFcn=PreScanBlockDeleteFcn;
      mask Help: eval('openHelp(222)')
      mask Display: image(imread('State.png'))
  STATE_HumanAnimated_1 : Subsystem  Tag=StateAnim  Priority=0  mask(PreScan Sink Block: StateAnim){x0=110.99077293275076, y0=72.719711441663208, z0=0.2, Roll0=0, Pitch0=0, Yaw0=256.6630859375, TimeStep=1/100, MWS=1.95}
      mask prompts: x0 "Ini x-position VEHICLE wrt GLOBAL axis system [m]"; y0 "Ini y-position VEHICLE wrt GLOBAL axis system [m]"; z0 "Ini z-position VEHICLE wrt GLOBAL axis system [m]"; Roll0 "Ini roll-angle BODY wrt GLOBAL axis system [rad]"; Pitch0 "Ini pitch-angle BODY wrt GLOBAL axis system [rad]"; Yaw0 "Ini yaw-angle BODY wrt GLOBAL axis system [rad]"; TimeStep "Time Step [s]"; MWS "Max Walking Speed [m/s]"
      mask help:
      | The Actor State contains a vector signal of size (9x1), containing the following signals:
      |
      | -  Position                  (x,y,z)                                     [m]
      | -  Velocity                  (vx,vy,vz)                               [m/s]
      | -  Angles                    (Roll, Pitch, Yaw)                   [rad]
      |
      | The Actor state is defined in the global axis system.
      | The state is superponed on the Initial position defined in the GUI.
      |
      | For more information, please click Help.
      settings: DeleteFcn=PreScanBlockDeleteFcn;
      mask Help: eval('openHelp(222)')
      mask Display: image(imread('StateAnim.png'))
  STATE_Mazda_RX8_2 : Subsystem  Tag=State  Priority=0  mask(PreScan Sink Block: State){x0=87.082992553710938, y0=70.1616928100586, z0=0.50999999046325684, Roll0=0, Pitch0=0, Yaw0=180, TimeStep=1/100}
      mask prompts: x0 "Ini x-position VEHICLE wrt GLOBAL axis system [m]"; y0 "Ini y-position VEHICLE wrt GLOBAL axis system [m]"; z0 "Ini z-position VEHICLE wrt GLOBAL axis system [m]"; Roll0 "Ini roll-angle BODY wrt VEHICLE axis system [deg]"; Pitch0 "Ini pitch-angle BODY wrt VEHICLE axis system [deg]"; Yaw0 "Ini yaw-angle VEHICLE wrt GLOBAL axis system [deg]"; TimeStep "Time Step [s]"
      mask help:
      | The Actor State contains a vector signal of size (9x1), containing the following signals:
      |
      | -  Position                  (x,y,z)                                     [m]
      | -  Velocity                  (vx,vy,vz)                               [m/s]
      | -  Angles                    (Roll, Pitch, Yaw)                   [rad]
      |
      | The Actor state is defined in the global axis system.
      | The state is superponed on the Initial position defined in the GUI.
      |
      | For more information, please click Help.
      settings: DeleteFcn=PreScanBlockDeleteFcn;
      mask Help: eval('openHelp(222)')
      mask Display: image(imread('State.png'))
  STATE_Mazda_RX8_3 : Subsystem  Tag=State  Priority=0  mask(PreScan Sink Block: State){x0=86.7197265625, y0=52.878681182861328, z0=0.50999999046325684, Roll0=0, Pitch0=0, Yaw0=0, TimeStep=1/100}
      mask prompts: x0 "Ini x-position VEHICLE wrt GLOBAL axis system [m]"; y0 "Ini y-position VEHICLE wrt GLOBAL axis system [m]"; z0 "Ini z-position VEHICLE wrt GLOBAL axis system [m]"; Roll0 "Ini roll-angle BODY wrt VEHICLE axis system [deg]"; Pitch0 "Ini pitch-angle BODY wrt VEHICLE axis system [deg]"; Yaw0 "Ini yaw-angle VEHICLE wrt GLOBAL axis system [deg]"; TimeStep "Time Step [s]"
      mask help:
      | The Actor State contains a vector signal of size (9x1), containing the following signals:
      |
      | -  Position                  (x,y,z)                                     [m]
      | -  Velocity                  (vx,vy,vz)                               [m/s]
      | -  Angles                    (Roll, Pitch, Yaw)                   [rad]
      |
      | The Actor state is defined in the global axis system.
      | The state is superponed on the Initial position defined in the GUI.
      |
      | For more information, please click Help.
      settings: DeleteFcn=PreScanBlockDeleteFcn;
      mask Help: eval('openHelp(222)')
      mask Display: image(imread('State.png'))
  STATE_Nissan_Cabstar_1 : Subsystem  Tag=State  Priority=0  mask(PreScan Sink Block: State){x0=114.25497436523437, y0=70.121936035156253, z0=0.87999999523162842, Roll0=0, Pitch0=0, Yaw0=180, TimeStep=1/100}
      mask prompts: x0 "Ini x-position VEHICLE wrt GLOBAL axis system [m]"; y0 "Ini y-position VEHICLE wrt GLOBAL axis system [m]"; z0 "Ini z-position VEHICLE wrt GLOBAL axis system [m]"; Roll0 "Ini roll-angle BODY wrt VEHICLE axis system [deg]"; Pitch0 "Ini pitch-angle BODY wrt VEHICLE axis system [deg]"; Yaw0 "Ini yaw-angle VEHICLE wrt GLOBAL axis system [deg]"; TimeStep "Time Step [s]"
      mask help:
      | The Actor State contains a vector signal of size (9x1), containing the following signals:
      |
      | -  Position                  (x,y,z)                                     [m]
      | -  Velocity                  (vx,vy,vz)                               [m/s]
      | -  Angles                    (Roll, Pitch, Yaw)                   [rad]
      |
      | The Actor state is defined in the global axis system.
      | The state is superponed on the Initial position defined in the GUI.
      |
      | For more information, please click Help.
      settings: DeleteFcn=PreScanBlockDeleteFcn;
      mask Help: eval('openHelp(222)')
      mask Display: image(imread('State.png'))
  STATE_Nissan_Cabstar_2 : Subsystem  Tag=State  Priority=0  mask(PreScan Sink Block: State){x0=122.5311279296875, y0=52.518203735351562, z0=0.87999999523162842, Roll0=0, Pitch0=0, Yaw0=0, TimeStep=1/100}
      mask prompts: x0 "Ini x-position VEHICLE wrt GLOBAL axis system [m]"; y0 "Ini y-position VEHICLE wrt GLOBAL axis system [m]"; z0 "Ini z-position VEHICLE wrt GLOBAL axis system [m]"; Roll0 "Ini roll-angle BODY wrt VEHICLE axis system [deg]"; Pitch0 "Ini pitch-angle BODY wrt VEHICLE axis system [deg]"; Yaw0 "Ini yaw-angle VEHICLE wrt GLOBAL axis system [deg]"; TimeStep "Time Step [s]"
      mask help:
      | The Actor State contains a vector signal of size (9x1), containing the following signals:
      |
      | -  Position                  (x,y,z)                                     [m]
      | -  Velocity                  (vx,vy,vz)                               [m/s]
      | -  Angles                    (Roll, Pitch, Yaw)                   [rad]
      |
      | The Actor state is defined in the global axis system.
      | The state is superponed on the Initial position defined in the GUI.
      |
      | For more information, please click Help.
      settings: DeleteFcn=PreScanBlockDeleteFcn;
      mask Help: eval('openHelp(222)')
      mask Display: image(imread('State.png'))
  STATE_Sphere_1 : Subsystem  Tag=State  Priority=0  mask(PreScan Sink Block: State){x0=134.499996185303, y0=66.6612396240235, z0=0.55, Roll0=0, Pitch0=0, Yaw0=180, TimeStep=1/100}
      mask prompts: x0 "Ini x-position VEHICLE wrt GLOBAL axis system [m]"; y0 "Ini y-position VEHICLE wrt GLOBAL axis system [m]"; z0 "Ini z-position VEHICLE wrt GLOBAL axis system [m]"; Roll0 "Ini roll-angle BODY wrt VEHICLE axis system [deg]"; Pitch0 "Ini pitch-angle BODY wrt VEHICLE axis system [deg]"; Yaw0 "Ini yaw-angle VEHICLE wrt GLOBAL axis system [deg]"; TimeStep "Time Step [s]"
      mask help:
      | The Actor State contains a vector signal of size (9x1), containing the following signals:
      |
      | -  Position                  (x,y,z)                                     [m]
      | -  Velocity                  (vx,vy,vz)                               [m/s]
      | -  Angles                    (Roll, Pitch, Yaw)                   [rad]
      |
      | The Actor state is defined in the global axis system.
      | The state is superponed on the Initial position defined in the GUI.
      |
      | For more information, please click Help.
      settings: DeleteFcn=PreScanBlockDeleteFcn;
      mask Help: eval('openHelp(222)')
      mask Display: image(imread('State.png'))
  STATE_Toyota_Previa_1 : Subsystem  Tag=State  Priority=0  mask(PreScan Sink Block: State){x0=129.08322906494141, y0=70.2, z0=0.70999997854232788, Roll0=0, Pitch0=0, Yaw0=180, TimeStep=1/100}
      mask prompts: x0 "Ini x-position VEHICLE wrt GLOBAL axis system [m]"; y0 "Ini y-position VEHICLE wrt GLOBAL axis system [m]"; z0 "Ini z-position VEHICLE wrt GLOBAL axis system [m]"; Roll0 "Ini roll-angle BODY wrt VEHICLE axis system [deg]"; Pitch0 "Ini pitch-angle BODY wrt VEHICLE axis system [deg]"; Yaw0 "Ini yaw-angle VEHICLE wrt GLOBAL axis system [deg]"; TimeStep "Time Step [s]"
      mask help:
      | The Actor State contains a vector signal of size (9x1), containing the following signals:
      |
      | -  Position                  (x,y,z)                                     [m]
      | -  Velocity                  (vx,vy,vz)                               [m/s]
      | -  Angles                    (Roll, Pitch, Yaw)                   [rad]
      |
      | The Actor state is defined in the global axis system.
      | The state is superponed on the Initial position defined in the GUI.
      |
      | For more information, please click Help.
      settings: DeleteFcn=PreScanBlockDeleteFcn;
      mask Help: eval('openHelp(222)')
      mask Display: image(imread('State.png'))
  STATE_Toyota_Previa_2 : Subsystem  Tag=State  Priority=0  mask(PreScan Sink Block: State){x0=115.06995391845703, y0=52.373069763183594, z0=0.70999997854232788, Roll0=0, Pitch0=0, Yaw0=0, TimeStep=1/100}
      mask prompts: x0 "Ini x-position VEHICLE wrt GLOBAL axis system [m]"; y0 "Ini y-position VEHICLE wrt GLOBAL axis system [m]"; z0 "Ini z-position VEHICLE wrt GLOBAL axis system [m]"; Roll0 "Ini roll-angle BODY wrt VEHICLE axis system [deg]"; Pitch0 "Ini pitch-angle BODY wrt VEHICLE axis system [deg]"; Yaw0 "Ini yaw-angle VEHICLE wrt GLOBAL axis system [deg]"; TimeStep "Time Step [s]"
      mask help:
      | The Actor State contains a vector signal of size (9x1), containing the following signals:
      |
      | -  Position                  (x,y,z)                                     [m]
      | -  Velocity                  (vx,vy,vz)                               [m/s]
      | -  Angles                    (Roll, Pitch, Yaw)                   [rad]
      |
      | The Actor state is defined in the global axis system.
      | The state is superponed on the Initial position defined in the GUI.
      |
      | For more information, please click Help.
      settings: DeleteFcn=PreScanBlockDeleteFcn;
      mask Help: eval('openHelp(222)')
      mask Display: image(imread('State.png'))
  STATE_Toyota_Previa_3 : Subsystem  Tag=State  Priority=0  mask(PreScan Sink Block: State){x0=94.289756774902344, y0=52.638362884521484, z0=0.70999997854232788, Roll0=0, Pitch0=0, Yaw0=0, TimeStep=1/100}
      mask prompts: x0 "Ini x-position VEHICLE wrt GLOBAL axis system [m]"; y0 "Ini y-position VEHICLE wrt GLOBAL axis system [m]"; z0 "Ini z-position VEHICLE wrt GLOBAL axis system [m]"; Roll0 "Ini roll-angle BODY wrt VEHICLE axis system [deg]"; Pitch0 "Ini pitch-angle BODY wrt VEHICLE axis system [deg]"; Yaw0 "Ini yaw-angle VEHICLE wrt GLOBAL axis system [deg]"; TimeStep "Time Step [s]"
      mask help:
      | The Actor State contains a vector signal of size (9x1), containing the following signals:
      |
      | -  Position                  (x,y,z)                                     [m]
      | -  Velocity                  (vx,vy,vz)                               [m/s]
      | -  Angles                    (Roll, Pitch, Yaw)                   [rad]
      |
      | The Actor state is defined in the global axis system.
      | The state is superponed on the Initial position defined in the GUI.
      |
      | For more information, please click Help.
      settings: DeleteFcn=PreScanBlockDeleteFcn;
      mask Help: eval('openHelp(222)')
      mask Display: image(imread('State.png'))
  STATE_Toyota_Previa_4 : Subsystem  Tag=State  Priority=0  mask(PreScan Sink Block: State){x0=122.11555480957031, y0=90.440689086914063, z0=0.70999997854232788, Roll0=0, Pitch0=0, Yaw0=90, TimeStep=1/100}
      mask prompts: x0 "Ini x-position VEHICLE wrt GLOBAL axis system [m]"; y0 "Ini y-position VEHICLE wrt GLOBAL axis system [m]"; z0 "Ini z-position VEHICLE wrt GLOBAL axis system [m]"; Roll0 "Ini roll-angle BODY wrt VEHICLE axis system [deg]"; Pitch0 "Ini pitch-angle BODY wrt VEHICLE axis system [deg]"; Yaw0 "Ini yaw-angle VEHICLE wrt GLOBAL axis system [deg]"; TimeStep "Time Step [s]"
      mask help:
      | The Actor State contains a vector signal of size (9x1), containing the following signals:
      |
      | -  Position                  (x,y,z)                                     [m]
      | -  Velocity                  (vx,vy,vz)                               [m/s]
      | -  Angles                    (Roll, Pitch, Yaw)                   [rad]
      |
      | The Actor state is defined in the global axis system.
      | The state is superponed on the Initial position defined in the GUI.
      |
      | For more information, please click Help.
      settings: DeleteFcn=PreScanBlockDeleteFcn;
      mask Help: eval('openHelp(222)')
      mask Display: image(imread('State.png'))
  STATE_Toyota_Yaris_1 : Subsystem  Tag=State  Priority=0  mask(PreScan Sink Block: State){x0=139.99999618530273, y0=63.161239624023438, z0=0.57, Roll0=0, Pitch0=0, Yaw0=180, TimeStep=1/100}
      mask prompts: x0 "Ini x-position VEHICLE wrt GLOBAL axis system [m]"; y0 "Ini y-position VEHICLE wrt GLOBAL axis system [m]"; z0 "Ini z-position VEHICLE wrt GLOBAL axis system [m]"; Roll0 "Ini roll-angle BODY wrt VEHICLE axis system [deg]"; Pitch0 "Ini pitch-angle BODY wrt VEHICLE axis system [deg]"; Yaw0 "Ini yaw-angle VEHICLE wrt GLOBAL axis system [deg]"; TimeStep "Time Step [s]"
      mask help:
      | The Actor State contains a vector signal of size (9x1), containing the following signals:
      |
      | -  Position                  (x,y,z)                                     [m]
      | -  Velocity                  (vx,vy,vz)                               [m/s]
      | -  Angles                    (Roll, Pitch, Yaw)                   [rad]
      |
      | The Actor state is defined in the global axis system.
      | The state is superponed on the Initial position defined in the GUI.
      |
      | For more information, please click Help.
      settings: DeleteFcn=PreScanBlockDeleteFcn;
      mask Help: eval('openHelp(222)')
      mask Display: image(imread('State.png'))
  Scope Collision Detections : Subsystem  Tag=Scope Collision Detections
      settings: DeleteFcn=PreScanBlockDeleteFcn;
      settings: OpenFcn=|
      | blockname=[get_param(gcb,'Parent'),'/',get_param(gcb,'Name')];
      | subblockname=[blockname,'/Collision Detections'];
      | open_system(subblockname);
      | close_system(blockname);
      mask Display:
      | plot([0.5 9.5 9.5 0.5 0.5],[5 5 9 9 5])
      | plot(0,0)
      | plot(10,10)
      | text(0,1,'P+')
  Scope Collision IDs : Subsystem  Tag=Scope Collision IDs
      settings: DeleteFcn=PreScanBlockDeleteFcn;
      settings: OpenFcn=|
      | blockname=[get_param(gcb,'Parent'),'/',get_param(gcb,'Name')];
      | subblockname=[blockname,'/Collision IDs'];
      | open_system(subblockname);
      | close_system(blockname);
      mask Display:
      | plot([0.5 9.5 9.5 0.5 0.5],[5 5 9 9 5])
      | plot(0,0)
      | plot(10,10)
      | text(0,1,'P+')
  SetActuators : Subsystem  Tag=SetActuators  Priority=1  mask(PreScan Simulation Core Block){TimeStep=1/100, NrOfActuators=572}
      mask prompts: TimeStep "Timestep [s]"; NrOfActuators "Number of actuator values"
      mask help:
      | Please do not remove this block from the PreScan compilation sheet,
      | as it contains essential configuration parameters for a PreScan simulation.
      settings: DeleteFcn=PreScanBlockDeleteFcn;
  SimCoreConfiguration : M-S-Function  Tag=SimCoreConfiguration  Description=8A5EF53B4861190E56FB66E044CDD90CE2A0C0441EB2C197D10D2452522F82BA  FunctionName=SimCoreBlock  Parameters=ExperimentXML PortsXML SimulationCore HostName CheckStart EnableLog RfR EnableGPUAccel ShowComputationTime  mask(PreScan Simulation Core Configurator){SimulationCore=NUTS, HostName=0, CheckStart=0, prescanversion='7.4.0', EnableLog=off, RfR=0, EnableGPUAccel=off, ShowComputationTime=off}
      mask prompts: SimulationCore "Simulation Core"; HostName "Simulation Host"; CheckStart "Show START Dialog"; prescanversion "PreScan Version"; EnableLog "Create TA Log"; RfR "Record for Replay"; EnableGPUAccel "Enable GPU Acceleration"; ShowComputationTime "Show ComputationTime Scope"
      mask help:
      | Please do not remove this block from the PreScan compilation sheet,
      | as it contains essential configuration parameter for a PreScan simulation.
      mask init:
      | model = bdroot;
      | ExperimentXML = [model(1:end-3) '.pex'];
      | PortsXML = [model '_ports.pcd'];
      settings: DeleteFcn=PreScanBlockDeleteFcn;  ModelCloseFcn=assignin('base',['model_closed_' bdroot],true);
      mask Help: eval('openHelp(812)')
      mask Display: image(imread('prescanlogo.ico'))
  SimCoreInfo : Subsystem  Tag=SimCoreInfo
  Sphere_1 : Subsystem  Tag=WorldObjectSubSystem  InitFcn=UniqueId = '237';
      mask Display: image(imread('Sphere.jpg'));color('white');text(0,0,' ID=68\n')
  Stop Simulation : Stop
  Subsystem : Subsystem
      mask Display: fprintf('CD');
  TIS_1 : S-Function  Priority=3  LoadFcn=load('PrescanScannerSensorData.mat');load('PrescanScannerSensorMessage.mat')  FunctionName=sfun_TISSensor  Parameters=timestepMask maxInputMessages maxOutputMessages sensorID detectableObjects  EnableBusSupport=off  mask{timestepMask=1/25, maxInputMessages=0, maxOutputMessages=32, sensorID=222, detectableObjects=32}
      mask prompts: timestepMask "MATLAB timestep:"; maxInputMessages "Max input messages:"; maxOutputMessages "Max output messages:"; sensorID "Sensor ID:"; detectableObjects "Max detectable objects:"
      mask help: TIS Sensor I/O
      mask Display: image(imread('TIS.png'))
  Toyota_Previa_1 : Subsystem  Tag=WorldObjectSubSystem  InitFcn=UniqueId = '24';
      mask Display: image(imread('Toyota_Previa.jpg'));color('white');text(0,0,' ID=11\n')
  Toyota_Previa_2 : Subsystem  Tag=WorldObjectSubSystem  InitFcn=UniqueId = '141';
      mask Display: image(imread('Toyota_Previa.jpg'));color('white');text(0,0,' ID=47\n')
  Toyota_Previa_3 : Subsystem  Tag=WorldObjectSubSystem  InitFcn=UniqueId = '142';
      mask Display: image(imread('Toyota_Previa.jpg'));color('white');text(0,0,' ID=48\n')
  Toyota_Previa_4 : Subsystem  Tag=WorldObjectSubSystem  InitFcn=UniqueId = '164';
      mask Display: image(imread('Toyota_Previa.jpg'));color('white');text(0,0,' ID=93\n')
  Toyota_Yaris_1 : Subsystem  Tag=WorldObjectSubSystem  InitFcn=UniqueId = '225';
      mask Display: image(imread('Toyota_Yaris.jpg'));color('white');text(0,0,' ID=32\n')
  VISULightSource_Audi_A8_1 : Subsystem  Tag=VisuLightSource  Priority=0
      settings: DeleteFcn=PreScanBlockDeleteFcn;
      mask Type: PreScan Sink Block: VisuLightSource
      mask Description:
      | The VisuLightSource block provides a way to animate Light Sources of the indicator, braking, fog and main lights of a vehicle.
      | 
      | For more information, please click Help.
      mask Help: eval('openHelp(223)')
      mask Display: image(imread('RearLight.png'))
  VISUTextureColor_Fiat_Bravo_1 : Subsystem  Tag=VisuTextureColor  Priority=0
      settings: DeleteFcn=PreScanBlockDeleteFcn;
      mask Type: PreScan Sink Block: VisuTextureColor
      mask Description:
      | The Texture Color block provides a way to adapt the color of a vehicle.
      | 
      | For more information, please click Help.
      mask Help: eval('openHelp(230)')
      mask Display: image(imread('TextureColor.png'))
  VISUTextureColor_Toyota_Previa_1 : Subsystem  Tag=VisuTextureColor  Priority=0
      settings: DeleteFcn=PreScanBlockDeleteFcn;
      mask Type: PreScan Sink Block: VisuTextureColor
      mask Description:
      | The Texture Color block provides a way to adapt the color of a vehicle.
      | 
      | For more information, please click Help.
      mask Help: eval('openHelp(230)')
      mask Display: image(imread('TextureColor.png'))
  VISUTextureColor_Toyota_Yaris_1 : Subsystem  Tag=VisuTextureColor  Priority=0
      settings: DeleteFcn=PreScanBlockDeleteFcn;
      mask Type: PreScan Sink Block: VisuTextureColor
      mask Description:
      | The Texture Color block provides a way to adapt the color of a vehicle.
      | 
      | For more information, please click Help.
      mask Help: eval('openHelp(230)')
      mask Display: image(imread('TextureColor.png'))
  VISUWheels_Audi_A8_1 : Subsystem  Tag=VisuWheels  Priority=0
      settings: DeleteFcn=PreScanBlockDeleteFcn;
      mask Type: PreScan Sink Block: VisuWheels
      mask Description:
      | The VisuWheels block provides a way to animate the wheels of a vehicle, with steering, rotation (because of velocity) and z-displacement.
      | 
      | For more information, please click Help.
      mask Help: eval('openHelp(223)')
      mask Display: image(imread('wheel.png'))
  VISUWheels_Ford_Fiesta_1 : Subsystem  Tag=VisuWheels  Priority=0
      settings: DeleteFcn=PreScanBlockDeleteFcn;
      mask Type: PreScan Sink Block: VisuWheels
      mask Description:
      | The VisuWheels block provides a way to animate the wheels of a vehicle, with steering, rotation (because of velocity) and z-displacement.
      | 
      | For more information, please click Help.
      mask Help: eval('openHelp(223)')
      mask Display: image(imread('wheel.png'))
  VISUWheels_Toyota_Yaris_1 : Subsystem  Tag=VisuWheels  Priority=0
      settings: DeleteFcn=PreScanBlockDeleteFcn;
      mask Type: PreScan Sink Block: VisuWheels
      mask Description:
      | The VisuWheels block provides a way to animate the wheels of a vehicle, with steering, rotation (because of velocity) and z-displacement.
      | 
      | For more information, please click Help.
      mask Help: eval('openHelp(223)')
      mask Display: image(imread('wheel.png'))
  tag scope: cd=global
  wires:
  Subsystem/1(cd_out) -> [cd], Stop Simulation/1
  CollisionDetection/1(U) -> Scope Collision IDs/1(In1)
  CollisionDetection/2(U1) -> Scope Collision Detections/1(In1), Subsystem/1(cd_in)
  BMW_X5_1/1(STATE_BMW_X5_1) -> STATE_BMW_X5_1/1(State)
  SELF_BMW_X5_1/1(U) -> BMW_X5_1/1(SELF_BMW_X5_1)
  BMW_Z3_1/1(STATE_BMW_Z3_1) -> STATE_BMW_Z3_1/1(State)
  SELF_BMW_Z3_1/1(U) -> BMW_Z3_1/1(SELF_BMW_Z3_1)
  Toyota_Previa_1/1(STATE_Toyota_Previa_1) -> STATE_Toyota_Previa_1/1(State)
  SELF_Toyota_Previa_1/1(U) -> Toyota_Previa_1/1(SELF_Toyota_Previa_1)
  Toyota_Previa_1/2(VISUTextureColor_Toyota_Previa_1) -> VISUTextureColor_Toyota_Previa_1/1(TextureColor)
  Nissan_Cabstar_1/1(STATE_Nissan_Cabstar_1) -> STATE_Nissan_Cabstar_1/1(State)
  SELF_Nissan_Cabstar_1/1(U) -> Nissan_Cabstar_1/1(SELF_Nissan_Cabstar_1)
  HumanAnimated_1/1(STATE_HumanAnimated_1) -> STATE_HumanAnimated_1/1(State)
  SELF_HumanAnimated_1/1(U) -> HumanAnimated_1/1(SELF_HumanAnimated_1)
  Mazda_RX8_2/1(STATE_Mazda_RX8_2) -> STATE_Mazda_RX8_2/1(State)
  SELF_Mazda_RX8_2/1(U) -> Mazda_RX8_2/1(SELF_Mazda_RX8_2)
  Fiat_Bravo_2/1(STATE_Fiat_Bravo_2) -> STATE_Fiat_Bravo_2/1(State)
  SELF_Fiat_Bravo_2/1(U) -> Fiat_Bravo_2/1(SELF_Fiat_Bravo_2)
  Toyota_Previa_2/1(STATE_Toyota_Previa_2) -> STATE_Toyota_Previa_2/1(State)
  SELF_Toyota_Previa_2/1(U) -> Toyota_Previa_2/1(SELF_Toyota_Previa_2)
  Toyota_Previa_3/1(STATE_Toyota_Previa_3) -> STATE_Toyota_Previa_3/1(State)
  SELF_Toyota_Previa_3/1(U) -> Toyota_Previa_3/1(SELF_Toyota_Previa_3)
  Mazda_RX8_3/1(STATE_Mazda_RX8_3) -> STATE_Mazda_RX8_3/1(State)
  SELF_Mazda_RX8_3/1(U) -> Mazda_RX8_3/1(SELF_Mazda_RX8_3)
  Nissan_Cabstar_2/1(STATE_Nissan_Cabstar_2) -> STATE_Nissan_Cabstar_2/1(State)
  SELF_Nissan_Cabstar_2/1(U) -> Nissan_Cabstar_2/1(SELF_Nissan_Cabstar_2)
  Toyota_Previa_4/1(STATE_Toyota_Previa_4) -> STATE_Toyota_Previa_4/1(State)
  SELF_Toyota_Previa_4/1(U) -> Toyota_Previa_4/1(SELF_Toyota_Previa_4)
  BMW_X5_2/1(STATE_BMW_X5_2) -> STATE_BMW_X5_2/1(State)
  SELF_BMW_X5_2/1(U) -> BMW_X5_2/1(SELF_BMW_X5_2)
  Audi_A8_1/1(STATE_Audi_A8_1) -> STATE_Audi_A8_1/1(State)
  SELF_Audi_A8_1/1(U) -> Audi_A8_1/1(SELF_Audi_A8_1)
  TIS_1/1 -> Audi_A8_1/2(TIS_1)
  CameraSensor_1/1(U1) -> Audi_A8_1/3(CameraSensor_1)
  Audi_A8_1/2(VISULightSource_Audi_A8_1) -> VISULightSource_Audi_A8_1/1(Lights)
  Audi_A8_1/3(VISUWheels_Audi_A8_1) -> VISUWheels_Audi_A8_1/1(Wheels)
  Toyota_Yaris_1/1(STATE_Toyota_Yaris_1) -> STATE_Toyota_Yaris_1/1(State)
  SELF_Toyota_Yaris_1/1(U) -> Toyota_Yaris_1/1(SELF_Toyota_Yaris_1)
  Toyota_Yaris_1/2(VISUTextureColor_Toyota_Yaris_1) -> VISUTextureColor_Toyota_Yaris_1/1(TextureColor)
  Toyota_Yaris_1/3(VISUWheels_Toyota_Yaris_1) -> VISUWheels_Toyota_Yaris_1/1(Wheels)
  Ford_Fiesta_1/1(STATE_Ford_Fiesta_1) -> STATE_Ford_Fiesta_1/1(State)
  SELF_Ford_Fiesta_1/1(U) -> Ford_Fiesta_1/1(SELF_Ford_Fiesta_1)
  Ford_Fiesta_1/2(VISUWheels_Ford_Fiesta_1) -> VISUWheels_Ford_Fiesta_1/1(Wheels)
  CarTrailer_SingleAxle_1/1(STATE_CarTrailer_SingleAxle_1) -> STATE_CarTrailer_SingleAxle_1/1(State)
  SELF_CarTrailer_SingleAxle_1/1(U) -> CarTrailer_SingleAxle_1/1(SELF_CarTrailer_SingleAxle_1)
  Sphere_1/1(STATE_Sphere_1) -> STATE_Sphere_1/1(State)
  SELF_Sphere_1/1(U) -> Sphere_1/1(SELF_Sphere_1)
  Fiat_Bravo_1/1(STATE_Fiat_Bravo_1) -> STATE_Fiat_Bravo_1/1(State)
  SELF_Fiat_Bravo_1/1(U) -> Fiat_Bravo_1/1(SELF_Fiat_Bravo_1)
  Fiat_Bravo_1/2(VISUTextureColor_Fiat_Bravo_1) -> VISUTextureColor_Fiat_Bravo_1/1(TextureColor)
  SetActuators/1(dummy) -> GetSensors/1(dummy)
